simulink model "MPCControllerIntegralAction"  (R2022a)
settings: Solver=ode4  StartTime=0.0  StopTime=inf  FixedStep=0.1  RelTol=1e-3
undefined symbols (not defined in the file or in its folder): A, B, C, D, K
settings Model: PacingRate=1000  Creator=Jan-Robin  LastModifiedBy=Jan-Robin

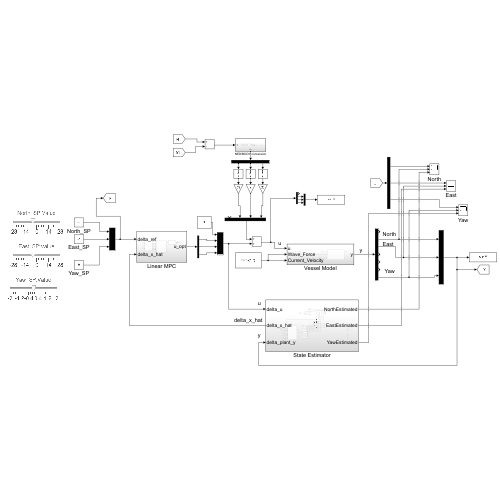
[thumbnail: Simulink's stored preview of the top-level diagram]
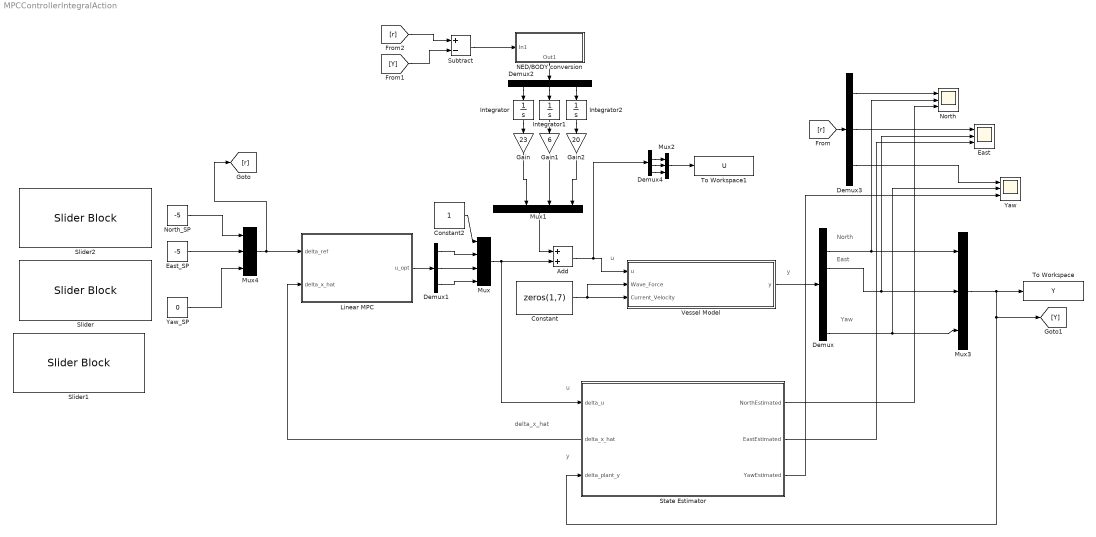
== system MPCControllerIntegralAction ==
  note: Yaw
  note: y
  note: East
  note: u
  note: u
  note: y
  note: North
  note: delta_x_hat
  Add : Sum
  Constant : Constant  Value=zeros(1,7)
  Constant2 : Constant
  Demux : Demux  Outputs=7
  Demux1 : Demux  Outputs=3
  Demux2 : Demux  Outputs=3
  Demux3 : Demux  Outputs=3
  Demux4 : Demux
  East : Scope  NumInputPorts=3
  East_SP : Constant  Value=-5
  Gain : Gain  Gain=23
  Gain1 : Gain  Gain=6
  Gain2 : Gain  Gain=20
  Integrator : Integrator
  Integrator1 : Integrator
  Integrator2 : Integrator
  Linear MPC : Subsystem
  Mux : Mux
  Mux1 : Mux
  Mux2 : Mux  Inputs=3
  Mux3 : Mux  Inputs=3
  Mux4 : Mux  Inputs=3
  NED/BODY conversion : Subsystem
      settings: PortSchema="{\"entries\":[{\"content\":{\"sides\":[{\"content\":{\"connectorIds\":[\"In1\"]},\"type\":\"ConnectorPlacement.EquallySpacedRectSide\",\"uuid\":\"1eb9fb5e-b235-4a22-912f-888b128d2d25\"},{\"content\":{\"connectorIds\":[],\"side\":\"RIGHT\"},\"type\":\"ConnectorPlacement.EquallySpacedRectSide\",\"uuid\":\"5813d27a-b72a-4c85-9394-e4af147ea912\"},{\"content\":{\"connectorIds\":[],\"side\":\"TOP\"},\"type\":\"ConnectorPlacement.EquallySpacedRectSide\",\"uuid\":\"5c3cc5a4-5ea7-4796-8384-52ad0a51e59e\"},{\"content\":{\"connectorIds\":[\"Out1\"],\"side\":\"BOTTOM\"},\"type\":\"ConnectorPlacement.EquallySpacedRectSide\",\"uuid\":\"71318ecd-9a69-4a48-91b3-40c3f31bc8c2\"}]},\"type\":\"ConnectorPlacement.EquallySpacedConnector\",\"uuid\":\"ac83cbd7-73fc-4253-a446-1ebb3357014a\"}],\"packageUris\":[\"http://schema.mathworks.com/mf0/Connector/R2020b\"],\"version\":\"1.0\"}"
  North : Scope  NumInputPorts=3
  North_SP : Constant  Value=-5
  Slider : SliderBlock  ScaleMin=-28  ScaleMax=28
  Slider1 : SliderBlock  ScaleMin=-2  ScaleMax=2
  Slider2 : SliderBlock  ScaleMin=-28  ScaleMax=28
  State Estimator : Subsystem
      settings: PortSchema="{\"entries\":[{\"content\":{\"sides\":[{\"content\":{\"connectorIds\":[\"In1\",\"Out4\",\"In2\"]},\"type\":\"ConnectorPlacement.EquallySpacedRectSide\",\"uuid\":\"9c8ac4e3-02eb-464a-9f84-8cc0f9418243\"},{\"content\":{\"connectorIds\":[\"Out1\",\"Out2\",\"Out3\"],\"side\":\"RIGHT\"},\"type\":\"ConnectorPlacement.EquallySpacedRectSide\",\"uuid\":\"66f11e56-0dca-41e5-b0a3-a654565c51d0\"},{\"content\":{\"connectorIds\":[],\"side\":\"TOP\"},\"type\":\"ConnectorPlacement.EquallySpacedRectSide\",\"uuid\":\"dd0d86d5-afb0-4c3e-a036-922a7e06e96c\"}]},\"type\":\"ConnectorPlacement.EquallySpacedConnector\",\"uuid\":\"affa5596-7398-454f-919c-bddd336a8178\"}],\"packageUris\":[\"http://schema.mathworks.com/mf0/Connector/R2020b\"],\"version\":\"1.0\"}"
  Subtract : Sum  Inputs=+-
  To Workspace : ToWorkspace  VariableName=Y  SampleTime=0.1
  To Workspace1 : ToWorkspace  VariableName=U  SampleTime=0.1
  Vessel Model : Subsystem
  Yaw : Scope  NumInputPorts=3
  Yaw_SP : Constant  Value=0
  wires:
  Demux1/1 -> Mux/2
  [r] -> Demux3/1
  Linear MPC/1(u_opt) -> Demux1/1
  Demux4/4 -> Mux2/3
  Demux/3 -> Mux3/2, East/2
  East_SP/1 -> Mux4/2
  Demux4/2 -> Mux2/1
  Demux3/3 -> Yaw/1
  State Estimator/4(delta_x_hat) -> Linear MPC/2(delta_x_hat)
  Demux1/3 -> Mux/4
  Yaw_SP/1 -> Mux4/3
  Demux/2 -> Mux3/1, North/2
  Vessel Model/1(y) -> Demux/1
  Constant2/1 -> Mux/1
  Mux3/1 -> To Workspace/1, State Estimator/2(delta_plant_y), [Y]
  Demux/7 -> Yaw/2, Mux3/3
  Demux4/3 -> Mux2/2
  North_SP/1 -> Mux4/1
  Mux4/1 -> [r], Linear MPC/1(delta_ref)
  State Estimator/3(YawEstimated) -> Yaw/3
  Mux2/1 -> To Workspace1/1
  Demux3/1 -> North/1
  State Estimator/2(EastEstimated) -> East/3
  State Estimator/1(NorthEstimated) -> North/3
  Mux/1 -> State Estimator/1(delta_u), Add/2
  Demux3/2 -> East/1
  Constant/1 -> Vessel Model/2(Wave_Force), Vessel Model/3(Current_Velocity)
  Demux1/2 -> Mux/3
  Demux2/1 -> Integrator/1
  Demux2/3 -> Integrator2/1
  Demux2/2 -> Integrator1/1
  Add/1 -> Demux4/1, Vessel Model/1(u)
  Mux1/1 -> Add/1
  Integrator/1 -> Gain/1
  Integrator1/1 -> Gain1/1
  Gain1/1 -> Mux1/3
  Gain/1 -> Mux1/2
  Subtract/1 -> NED/BODY conversion/1(In1)
  NED/BODY conversion/1(Out1) -> Demux2/1
  Integrator2/1 -> Gain2/1
  Gain2/1 -> Mux1/4
  [Y] -> Subtract/2
  [r] -> Subtract/1

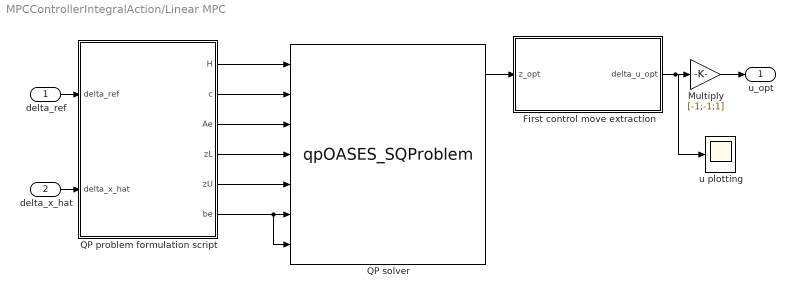
== system MPCControllerIntegralAction/Linear MPC ==
  delta_ref : Inport
  delta_x_hat : Inport  Port=2
  First control move extraction : MATLAB Function  TreatAsAtomicUnit=on
  Multiply : Gain  Gain=[-1;-1;1]
  QP problem formulation script : MATLAB Function  TreatAsAtomicUnit=on
  QP solver : S-Function  FunctionName=qpOASES_SQProblem  SFunctionDeploymentMode=off  EnableBusSupport=off
  u plotting : Scope
  u_opt : Outport
  wires:
  QP solver/1 -> First control move extraction/1(z_opt)
  delta_x_hat/1 -> QP problem formulation script/2(delta_x_hat)
  delta_ref/1 -> QP problem formulation script/1(delta_ref)
  QP problem formulation script/1(H) -> QP solver/1
  QP problem formulation script/2(c) -> QP solver/2
  QP problem formulation script/3(Ae) -> QP solver/3
  QP problem formulation script/4(zL) -> QP solver/4
  QP problem formulation script/5(zU) -> QP solver/5
  QP problem formulation script/6(be) -> QP solver/7, QP solver/6
  First control move extraction/1(delta_u_opt) -> Multiply/1, u plotting/1
  Multiply/1 -> u_opt/1

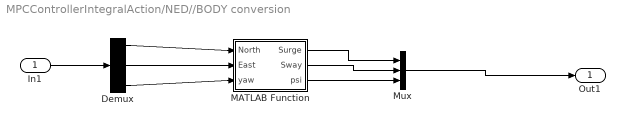
== system MPCControllerIntegralAction/NED//BODY conversion ==
  In1 : Inport
  Demux : Demux  Outputs=3
  MATLAB Function : MATLAB Function  TreatAsAtomicUnit=on
  Mux : Mux  Inputs=3
  Out1 : Outport
  wires:
  In1/1 -> Demux/1
  Demux/1 -> MATLAB Function/1(North)
  Demux/3 -> MATLAB Function/3(yaw)
  Demux/2 -> MATLAB Function/2(East)
  MATLAB Function/1(Surge) -> Mux/1
  MATLAB Function/2(Sway) -> Mux/2
  MATLAB Function/3(psi) -> Mux/3
  Mux/1 -> Out1/1

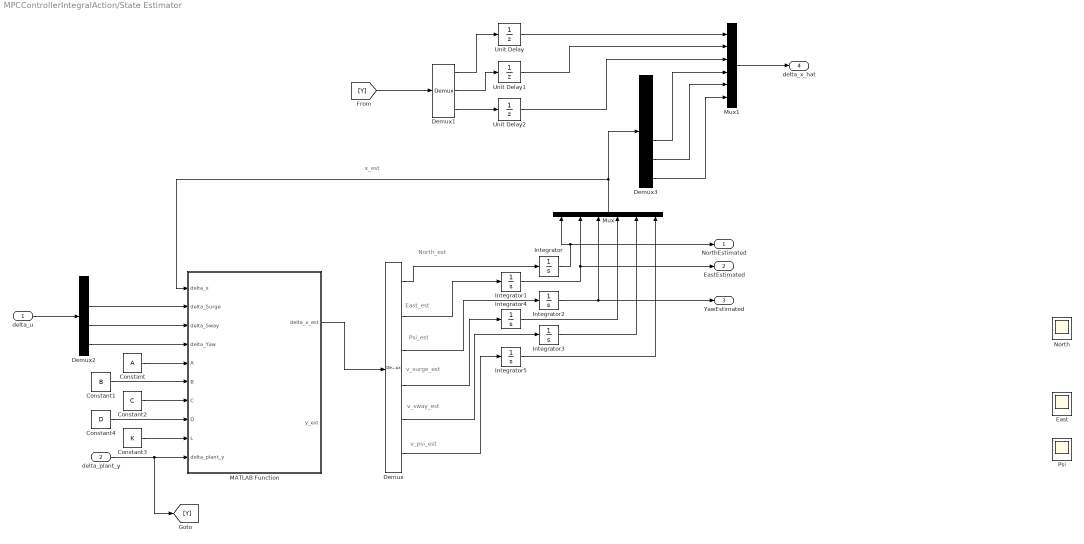
== system MPCControllerIntegralAction/State Estimator ==
  note: x_est
  note: v_psi_est
  note: v_sway_est
  note: v_surge_est
  note: Psi_est
  note: East_est
  note: North_est
  delta_u : Inport
  delta_plant_y : Inport  Port=2
  Constant : Constant  Value=A
  Constant1 : Constant  Value=B
  Constant2 : Constant  Value=C
  Constant3 : Constant  Value=K
  Constant4 : Constant  Value=D
  Demux : Demux  Outputs=6
  Demux1 : Demux  Outputs=3
  Demux2 : Demux
  Demux3 : Demux  Outputs=6
  East : Scope  NumInputPorts=3
  Integrator : Integrator  LimitOutput=on  UpperSaturationLimit=100  LowerSaturationLimit=-100
  Integrator1 : Integrator  LimitOutput=on  UpperSaturationLimit=100  LowerSaturationLimit=-100
  Integrator2 : Integrator  InitialCondition=-0.0005  UpperSaturationLimit=0.4  LowerSaturationLimit=-0.4
  Integrator3 : Integrator  InitialCondition=0.0067  UpperSaturationLimit=4  LowerSaturationLimit=-4
  Integrator4 : Integrator  InitialCondition=0.1385  UpperSaturationLimit=4  LowerSaturationLimit=-4
  Integrator5 : Integrator  InitialCondition=-0.0017  UpperSaturationLimit=0.2  LowerSaturationLimit=-0.2
  MATLAB Function : MATLAB Function  TreatAsAtomicUnit=on
  Mux : Mux  Inputs=6
  Mux1 : Mux  Inputs=6
  North : Scope  NumInputPorts=3
  Psi : Scope  NumInputPorts=2
  Unit Delay : UnitDelay  SampleTime=-1  HasFrameUpgradeWarning=on
  Unit Delay1 : UnitDelay  SampleTime=-1  HasFrameUpgradeWarning=on
  Unit Delay2 : UnitDelay  SampleTime=-1  HasFrameUpgradeWarning=on
  NorthEstimated : Outport
  EastEstimated : Outport  Port=2
  YawEstimated : Outport  Port=3
  delta_x_hat : Outport  Port=4
  wires:
  Demux2/3 -> MATLAB Function/3(delta_Sway)
  Demux2/4 -> MATLAB Function/4(delta_Yaw)
  delta_plant_y/1 -> [Y], MATLAB Function/10(delta_plant_y)
  Constant2/1 -> MATLAB Function/7(C)
  Constant3/1 -> MATLAB Function/9(L)
  MATLAB Function/1(delta_x_est) -> Demux/1
  Demux/1 -> Integrator/1
  Demux/2 -> Integrator1/1
  Demux/3 -> Integrator2/1
  Demux/4 -> Integrator4/1
  Demux/5 -> Integrator3/1
  Demux/6 -> Integrator5/1
  Integrator/1 -> Mux/1, NorthEstimated/1
  Integrator1/1 -> EastEstimated/1, Mux/2
  Integrator2/1 -> YawEstimated/1, Mux/3
  Integrator4/1 -> Mux/4
  Integrator3/1 -> Mux/5
  Integrator5/1 -> Mux/6
  Constant/1 -> MATLAB Function/5(A)
  Constant1/1 -> MATLAB Function/6(B)
  Constant4/1 -> MATLAB Function/8(D)
  Mux/1 -> Demux3/1, MATLAB Function/1(delta_x)
  delta_u/1 -> Demux2/1
  Demux2/2 -> MATLAB Function/2(delta_Surge)
  Demux3/4 -> Mux1/4
  Demux3/5 -> Mux1/5
  Demux3/6 -> Mux1/6
  Mux1/1 -> delta_x_hat/1
  Demux1/1 -> Unit Delay/1
  Unit Delay/1 -> Mux1/1
  Demux1/2 -> Unit Delay1/1
  Demux1/3 -> Unit Delay2/1
  Unit Delay1/1 -> Mux1/2
  Unit Delay2/1 -> Mux1/3
  [Y] -> Demux1/1

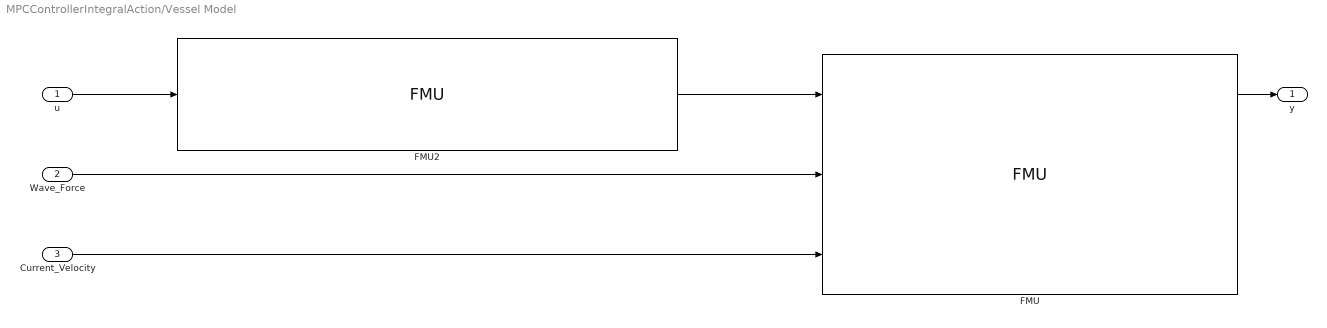
== system MPCControllerIntegralAction/Vessel Model ==
  u : Inport
  Wave_Force : Inport  Port=2
  Current_Velocity : Inport  Port=3
  FMU : FMU  FMUName=VesselModel.fmu  FMUMode=CoSimulation  Axc=106.0  Ayc=419.0  Bv_0_=44000.0  Bv_1_=0.0  Bv_2_=0.0  Bv_3_=0.0  Bv_4_=0.0  Bv_5_=0.0  Bv_6_=0.0  Bv_7_=177000.0  Bv_8_=0.0  Bv_9_=0.0  Bv_10_=0.0  Bv_11_=0.0  Bv_12_=0.0  Bv_13_=0.0  Bv_14_=0.0  Bv_15_=0.0  Bv_16_=0.0  Bv_17_=0.0  Bv_18_=0.0  Bv_19_=0.0  Bv_20_=0.0  Bv_21_=686000.0  Bv_22_=0.0  Bv_23_=0.0  Bv_24_=0.0  Bv_25_=0.0  Bv_26_=0.0  Bv_27_=0.0  Bv_28_=0.0  Bv_29_=0.0  Bv_30_=0.0  Bv_31_=0.0  Bv_32_=0.0  Bv_33_=0.0  Bv_34_=0.0  Bv_35_=1.0259E+7  Cx=1.0  Cy=0.7812  Dp_0_=5300.0  Dp_1_=0.0  Dp_2_=0.0  Dp_3_=0.0  Dp_4_=0.0  Dp_5_=0.0  Dp_6_=0.0  Dp_7_=21100.0  Dp_8_=0.0  Dp_9_=-20300.0  Dp_10_=0.0  Dp_11_=294000.0  Dp_12_=0.0  Dp_13_=0.0  Dp_14_=1900.0  Dp_15_=0.0  Dp_16_=-68400.0  Dp_17_=0.0  Dp_18_=0.0  Dp_19_=-20300.0  Dp_20_=0.0  Dp_21_=7600.0  Dp_22_=0.0  Dp_23_=-201300.0  Dp_24_=0.0  Dp_25_=0.0  Dp_26_=-68400.0  Dp_27_=0.0  Dp_28_=819700.0  Dp_29_=0.0  Dp_30_=0.0  Dp_31_=294000.0  Dp_32_=0.0  Dp_33_=-201300.0  Dp_34_=0.0  Dp_35_=1.8944E+6  G_0_=0.0  G_1_=0.0  G_2_=0.0  G_3_=0.0  G_4_=0.0  G_5_=0.0  G_6_=0.0  G_7_=0.0  G_8_=0.0  G_9_=0.0  G_10_=0.0  G_11_=0.0  G_12_=0.0  G_13_=0.0  G_14_=2.44E+6  G_15_=0.0  G_16_=1.78E+6  G_17_=0.0  G_18_=0.0  G_19_=0.0  G_20_=0.0  G_21_=5.11E+6  G_22_=0.0  G_23_=0.0  G_24_=0.0  G_25_=0.0  G_26_=1.78E+6  G_27_=0.0  G_28_=1.2737E+8  G_29_=0.0  G_30_=0.0  G_31_=0.0  G_32_=0.0  G_33_=0.0  G_34_=0.0  G_35_=0.0  Lpp=28.9  Minv_0_=1.268E-6  Minv_1_=0.0  Minv_2_=0.0  Minv_3_=0.0  Minv_4_=0.0  Minv_5_=0.0  Minv_6_=0.0  Minv_7_=1.083E-6  Minv_8_=0.0  Minv_9_=1.2E-8  Minv_10_=0.0  Minv_11_=1.0E-9  Minv_12_=0.0  Minv_13_=0.0  Minv_14_=5.9200000000000011E-7  Minv_15_=0.0  Minv_16_=-1.3E-8  Minv_17_=0.0  Minv_18_=0.0  Minv_19_=1.2E-8  Minv_20_=0.0  Minv_21_=1.0000000000000001E-7  Minv_22_=0.0  Minv_23_=-1.0E-9  Minv_24_=0.0  Minv_25_=0.0  Minv_26_=-1.3E-8  Minv_27_=0.0  Minv_28_=1.2E-8  Minv_29_=0.0  Minv_30_=0.0  Minv_31_=1.0E-9  Minv_32_=0.0  Minv_33_=-1.0E-9  Minv_34_=0.0  Minv_35_=2.0E-8  N=20.0  X_DOF_DP_model_Integrator1__InitialCondition_0_=0.0  X_DOF_DP_model_Integrator1__InitialCondition_1_=0.0  X_DOF_DP_model_Integrator1__InitialCondition_2_=0.0  X_DOF_DP_model_Integrator1__InitialCondition_3_=0.0  X_DOF_DP_model_Integrator1__InitialCondition_4_=0.0  X_DOF_DP_model_Integrator1__InitialCondition_5_=0.0  X_DOF_DP_model_Integrator2_InitialCondition_0_=0.0  X_DOF_DP_model_Integrator2_InitialCondition_1_=0.0  X_DOF_DP_model_Integrator2_InitialCondition_2_=0.0  X_DOF_DP_model_Integrator2_InitialCondition_3_=0.0  X_DOF_DP_model_Integrator2_InitialCondition_4_=0.0  X_DOF_DP_model_Integrator2_InitialCondition_5_=0.0  X_DOF_DP_model_Rotate_yaw_T_Constant_Value=0.0  X_DOF_DP_model_Rotate_yaw_T_psi_Value=0.0  X_DOF_DP_model_X_DOF_transformation_Euler_angles_to_att=0.0  X_DOF_DP_model_X_DOF_transformation_Euler_angles_to_att_2=1.0  X_DOF_DP_model_zero_Value=0.0  rho=1025.0  mask(VesselModel [Co-Simulation, v2.0]){}
  FMU2 : FMU  FMUName=ThrusterDynamics.fmu  FMUMode=CoSimulation  Heave_Thrust=struct('Value',0.0)  Merge1=struct('InitialOutput',0.0)  Pitch_Thrust=struct('Value',0.0)  Roll_Thrust=struct('Value',0.0)  Thruster_Dynamics=struct('Surge_Thrust_Dynamics',struct('A',-0.2,'C',0.2),'Sway_Thrust_Dynamics',struct('A',-0.2,'C',0.2),'Yaw_Thrust_Dynamics',struct('A',-0.2,'C',0.2))  enableDynamics=on  enableSaturation=on  maxThrust=[1.0E+10,1.0E+10,1.0E+11]  mask(ThrusterDynamics [Co-Simulation, v2.0]){}
  y : Outport
  wires:
  u/1 -> FMU2/1
  FMU2/1 -> FMU/1
  FMU/1 -> y/1
  Wave_Force/1 -> FMU/2
  Current_Velocity/1 -> FMU/3

== matlab function MPCControllerIntegralAction/Linear MPC/First control move extraction ==
  data: z_opt input; delta_u_opt output
function delta_u_opt = fcn(z_opt)
%no need for the control moves for the whole prediction horizon, selecting
%only the first.
delta_u_opt = z_opt(1:3);

== matlab function MPCControllerIntegralAction/Linear MPC/QP problem formulation script ==
  data: delta_ref input; delta_x_hat input; H output; c output; Ae output; zL output; zU output; be output; A parameter; B parameter; C parameter
function [H, c, Ae, zL, zU, be] = QP_formulation(delta_ref, delta_x_hat,A, B, C)

%A=Ad; B=Bd; C=Cd;

%Discrete time model is imported from 
%The system identification part. 

N = 20;                         %Prediction horizon length
Q = diag([4e4 9e4 8e4]);       %Weighting matrix for the error
P = diag([1e-6 1e-6 1e-6]); % Weighting matrix for the input

%%Q = diag([1 1 1 ]);       %Weighting matrix for the error
%P = 1e-3;                      % Weighting matrix for the input


x0=delta_x_hat;


r=[ones(1, N).*delta_ref(1);
    ones(1,N).*delta_ref(2);
    ones(1,N).*delta_ref(3)];  %make reference for the whole prediction lenght

%Build the QP problem
%Standard QP formulation
nx = size(A, 1); nu = size(B, 2); ny=size(C, 1); nz = N*(nx+nu+2*ny);

% Building H matrices
H11 = kron(eye(N),P);
H22= zeros(N*nx, N*nx);
H33 = kron(eye(N),Q);
H44 = zeros(N*ny, N*ny);
H_mat = blkdiag(H11,H22,H33,H44);

%qpOASES does not support matrices, but only vectors. Stacking collumn wise
H = H_mat(:);
c= zeros(nz, 1);

%Making the constraints
Ae1u = -kron(eye(N),B);
Ae1x = eye(N*nx)-kron(diag(ones(N-abs(-1),1),-1),A);
Ae1e = zeros(N*nx,N*ny);
Ae1y = zeros(N*nx,N*ny);
be1  =[A*x0;zeros((N-1)*nx,1)];

Ae2u = zeros(N*ny,N*nu);
Ae2x = -kron(eye(N),C);
Ae2e = zeros(N*ny,N*ny);
Ae2y = eye(N*ny);
be2 = zeros(N*ny, 1);

Ae3u = zeros(N*ny,N*nu);
Ae3x = zeros(N*ny,N*nx);
Ae3e = eye(N*ny);
Ae3y = eye(N*ny);
be3 = reshape(r, N*ny,1);

Ae_mat =[Ae1u Ae1x Ae1e Ae1y;
    Ae2u Ae2x Ae2e Ae2y;
    Ae3u Ae3x Ae3e Ae3y]; 

%qpOASES does not support matrices, but only vectors. Stacking collumn wise
Ae=Ae_mat(:);
be=[be1; be2; be3];

%bounds to be inserted when testing is complete
%Building bounds

zL = (-inf*ones(nz,1));
zU= (inf*ones(nz,1));
%  zL = [zeros(N*nu,1);-inf*ones(nz-N*nu-N*nx-N*ny,1);zeros(nz-N*ny,0)];
%  zU = [3*ones(N*nu,1);inf*ones(nz-N*nu-N*nx-N*ny,1);zeros(nz-N*ny,0)];

%  zL = [zeros(N*nu,1);-inf*ones(nz-N*nu,1)];
%  zU = [3*ones(N*nu,1);inf*ones(nz-N*nu,1)];

== matlab function MPCControllerIntegralAction/NED//BODY conversion/MATLAB Function ==
  data: North input; Surge output; East input; yaw input; Sway output; psi output
function [Surge, Sway, psi]= fcn(North, East, yaw)

%North - coordinates in north
%East - coordinates in east
%yaw - angle in radians

%Correcting variable name
psi = yaw;

%rotational matrix without Down
R_psi = [cos(psi), -sin(psi);
    sin(psi), cos(psi)];

%NED coordinates
P_NED = [North;East];

%Computing Body coordinates
P_body = R_psi*P_NED;

%Extract Surge and Sway components.
Surge = P_body(1);
Sway = P_body(2);

== matlab function MPCControllerIntegralAction/State Estimator/MATLAB Function ==
  data: delta_x input; delta_x_est output; delta_Surge input; delta_Sway input; delta_Yaw input; A input; B input; C input; D input; L input; delta_plant_y input; y_est output
function [delta_x_est,y_est]= state_estimator(delta_x, delta_Surge, delta_Sway, delta_Yaw,A, B,C, D,L,delta_plant_y)

%y_est = C*delta_x+D*[delta_Surge;delta_Sway;delta_Yaw];
y_est = C*delta_x;
delta_x_est = A*delta_x +B*[delta_Surge;delta_Sway;delta_Yaw] + L*(delta_plant_y-y_est);
